simulink model "MIL_2018"  (R2018a)
settings: Solver=FixedStepDiscrete  StartTime=0.0  StopTime=49  FixedStep=1  MaxStep=1  RelTol=1e-3
undefined symbols (not defined in the file or in its folder): sigbuilder_block
settings Model: DataDictionary=Als_dd.sldd  Creator=Pratik shinde  LastModifiedBy=Pratik shinde
settings DataIOCC: ReturnWorkspaceOutputs=on
settings OptimizationCC: DefaultParameterBehavior=Inlined  EnhancedBackFolding=on  PassReuseOutputArgsAs=Individual arguments  ZeroExternalMemoryAtStartup=off  ZeroInternalMemoryAtStartup=off  OptimizeBlockOrder=speed  DifferentSizesBufferReuse=on  OptimizationCustomize=off
settings DebuggingCC: ParameterTunabilityLossMsg=error  ModelReferenceSymbolNameMessage=none
settings SFSimCC: SimUseLocalCustomCode=on  MATLABDynamicMemAlloc=off
settings RTWCC: SystemTargetFile=ert.tlc  GenCodeOnly=on  TemplateMakefile=ert_default_tmf  GenerateReport=on  RTWUseLocalCustomCode=on  IncludeHyperlinkInReport=on  LaunchReport=on  GenerateTraceInfo=on  GenerateTraceReport=on  GenerateTraceReportSl=on  GenerateTraceReportSf=on  GenerateTraceReportEml=on  GenerateWebview=on
settings CodeAppCC: ForceParamTrailComments=on  IgnoreCustomStorageClasses=off  OperatorAnnotations=on  SimulinkDataObjDesc=on  SFDataObjDesc=on  InsertBlockDesc=on
settings ERTTargetCC: TargetLangStandard=C99 (ISO)  GenerateSampleERTMain=on  InlinedParameterPlacement=NonHierarchical  ERTCustomFileTemplate=example_file_process.tlc
settings ConfigComp: CovMetricSettings=dcmw  CovHtmlReporting=on  DVTestSuiteOptimization=CombinedObjectives (Nonlinear Extended)  DVDetectOutOfBounds=on

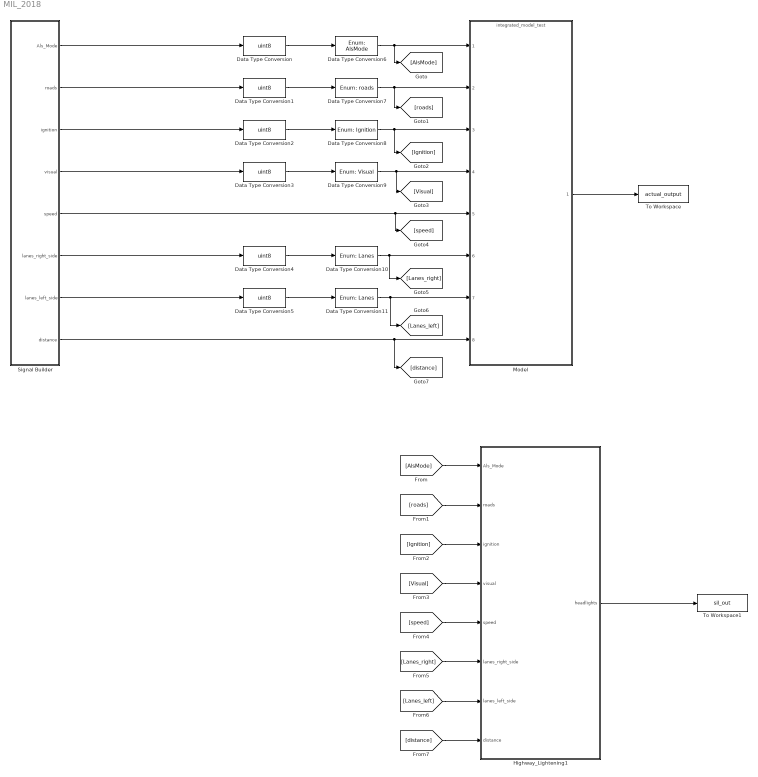
== system MIL_2018 ==
  Data Type Conversion{,1..5} (6 alike) : DataTypeConversion  OutDataTypeStr=uint8  SaturateOnIntegerOverflow=on  LockScale=on
  Data Type Conversion10 : DataTypeConversion  OutDataTypeStr=Enum: Lanes  SaturateOnIntegerOverflow=on  LockScale=on
  Data Type Conversion11 : DataTypeConversion  OutDataTypeStr=Enum: Lanes  SaturateOnIntegerOverflow=on  LockScale=on
  Data Type Conversion6 : DataTypeConversion  OutDataTypeStr=Enum: AlsMode  SaturateOnIntegerOverflow=on  LockScale=on
  Data Type Conversion7 : DataTypeConversion  OutDataTypeStr=Enum: roads  SaturateOnIntegerOverflow=on  LockScale=on
  Data Type Conversion8 : DataTypeConversion  OutDataTypeStr=Enum: Ignition  SaturateOnIntegerOverflow=on  LockScale=on
  Data Type Conversion9 : DataTypeConversion  OutDataTypeStr=Enum: Visual  SaturateOnIntegerOverflow=on  LockScale=on
  Highway_Lightening1 : Subsystem
      mask help: Simulink:masks:GenSFuncDesc_MD
      mask Help: eval('feval(''rtwprivate'',''rtwhelpview'',''rtw_sfcn_block'')');
  Model : ModelReference  ModelNameDialog=integrated_model_test.slx  SimulationMode=Normal  ModelReferenceVersion=1.36
  Signal Builder : Subsystem  Tag=STV Subsys  LoadFcn=sigbuilder_block('load');  StartFcn=sigbuilder_block('start');  StopFcn=sigbuilder_block('stop');  ClipboardFcn=sigbuilder_block('clipboard');  mask(Sigbuilder block){tuvar=[0:10]}
      mask help: Simulink:masks:SigbuilderBlock_MD
      mask init:
      | if ~strcmp(get_param(bdroot(gcbh),'SimulationStatus'),'stopped') tuvar = sigbuilder_block('maskInit'); end
      settings: CopyFcn=sigbuilder_block('copy');  DeleteFcn=sigbuilder_block('delete');  ModelCloseFcn=sigbuilder_block('modelClose');  PreSaveFcn=sigbuilder_block('preSave');  PauseFcn=sigbuilder_block('pause');  ContinueFcn=sigbuilder_block('continue');  NameChangeFcn=sigbuilder_block('namechange');  OpenFcn=sigbuilder_block('open',[437.6 199.2 550.4 400 ]);  CloseFcn=sigbuilder_block('close');
      mask Display: plot(0, 0, 100, 100,[2, 2, 32, 32, 2], [68, 8, 8, 68, 68],[32, 2], [38, 38], [32, 19, 2],[53, 60, 44], [32, 17, 17, 2],[16, 16, 31, 31]);txt = getActiveGroup(gcbh);text(2, 100, txt,'verticalAlignment', 'top');
  To Workspace : ToWorkspace  VariableName=actual_output  SaveFormat=Timeseries  SampleTime=-1
  To Workspace1 : ToWorkspace  VariableName=sil_out  SaveFormat=Timeseries  SampleTime=-1
  wires:
  Signal Builder/2(roads) -> Data Type Conversion1/1
  Signal Builder/3(ignition) -> Data Type Conversion2/1
  Signal Builder/4(visual) -> Data Type Conversion3/1
  Signal Builder/5(speed) -> [speed], Model/5
  Signal Builder/7(lanes_left_side) -> Data Type Conversion5/1
  Signal Builder/8(distance) -> [distance], Model/8
  Signal Builder/6(lanes_right_side) -> Data Type Conversion4/1
  Data Type Conversion/1 -> Data Type Conversion6/1
  Data Type Conversion1/1 -> Data Type Conversion7/1
  Data Type Conversion2/1 -> Data Type Conversion8/1
  Data Type Conversion3/1 -> Data Type Conversion9/1
  Data Type Conversion4/1 -> Data Type Conversion10/1
  Data Type Conversion5/1 -> Data Type Conversion11/1
  Data Type Conversion6/1 -> [AlsMode], Model/1
  Data Type Conversion7/1 -> [roads], Model/2
  Data Type Conversion8/1 -> [Ignition], Model/3
  Data Type Conversion9/1 -> [Visual], Model/4
  Data Type Conversion10/1 -> Model/6, [Lanes_right]
  Data Type Conversion11/1 -> Model/7, [Lanes_left]
  Model/1 -> To Workspace/1
  Signal Builder/1(Als_Mode) -> Data Type Conversion/1
  Highway_Lightening1/1(headlights) -> To Workspace1/1
  [AlsMode] -> Highway_Lightening1/1(Als_Mode)
  [roads] -> Highway_Lightening1/2(roads)
  [Ignition] -> Highway_Lightening1/3(ignition)
  [Visual] -> Highway_Lightening1/4(visual)
  [speed] -> Highway_Lightening1/5(speed)
  [Lanes_left] -> Highway_Lightening1/7(lanes_left_side)
  [distance] -> Highway_Lightening1/8(distance)
  [Lanes_right] -> Highway_Lightening1/6(lanes_right_side)

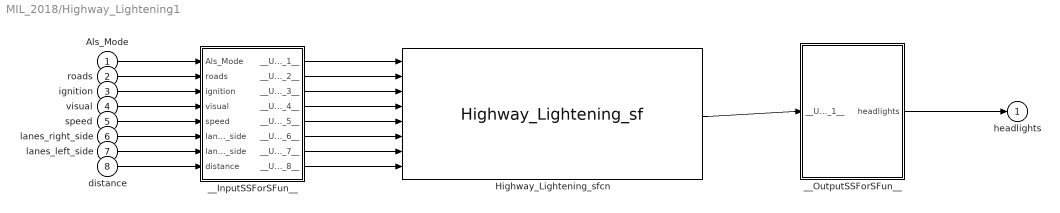
== system MIL_2018/Highway_Lightening1 ==
  Als_Mode : Inport
  roads : Inport  Port=2
  ignition : Inport  Port=3
  visual : Inport  Port=4
  speed : Inport  Port=5
  lanes_right_side : Inport  Port=6
  lanes_left_side : Inport  Port=7
  distance : Inport  Port=8
  Highway_Lightening_sfcn : S-Function  FunctionName=Highway_Lightening_sf  SFunctionModules=""  SFunctionDeploymentMode=off  EnableBusSupport=off  mask{rtw_sf_name=Highway_Lightening_sf, showVar=off}
      mask prompts: rtw_sf_name "Simulink:masks:GenSFuncName_MP"; showVar "Simulink:masks:GenSFuncShowModuleList_MP"
      mask help: Simulink:masks:GenSFuncDesc_MD
      mask init:
      | displist = '';
      | if ~strcmp(get_param(gcb, 'FunctionName'), rtw_sf_name);
      |   set_param(gcb, 'FunctionName', rtw_sf_name);
      | end
      | % Check if we are generating code
      | rtw_mode = false;
      | if strcmpi(get_param(bdroot(gcb),'SimulationStatus'),'Initializing')
      | 	rtw_mode = strcmpi(get_param(bdroot(gcb),'BuildingRTWCode'),'on') && ...
      | 		~strcmpi(get_param(bdroot(gcb),'TargetStyle'),'SimulationTarget');
      | end
      | if showVar || rtw_mode
      | 	if exist('rtwsfunc') == 2 | exist('rtwsfunc') == 6
      | 		tmplist = rtwsfunc(rtw_sf_name,gcb);
      | 		tmplist = DAStudio.message('Simulink:masks:GenSFuncListOfModules_IC', tmplist);
      | 	elseif showVar
      | 		tmplist1 = DAStudio.message('Simulink:masks:GenSFuncListOfModules_IC', '');
      |         tmplist2 = DAStudio.message('Simulink:masks:GenSFuncNotLicensed_IC');
      |         tmplist = [tmplist1 tmplist2];
      |  	end
      | end
      | if showVar
      |   displist = tmplist;
      | end
      settings: CopyFcn=|
      | if ~strcmp(get_param(gcb,'Linkstatus'),'none') && ...
      | ~strcmp(get_param(gcb,'Linkstatus'),'implicit')
      |   set_param(gcb,'LinkStatus','none');
      | end
      mask Help: eval('feval(''rtwprivate'',''rtwhelpview'',''rtw_sfcn_block'')');
      mask Display:
      | port_label('input',1,'Als_Mode');
      | port_label('input',2,'roads');
      | port_label('input',3,'ignition');
      | port_label('input',4,'visual');
      | port_label('input',5,'speed');
      | port_label('input',6,'lanes_right_side');
      | port_label('input',7,'lanes_left_side');
      | port_label('input',8,'distance');
      | port_label('output',1,'headlights');
  __InputSSForSFun__ : Subsystem
  __OutputSSForSFun__ : Subsystem
  headlights : Outport
  wires:
  __OutputSSForSFun__/1(headlights) -> headlights/1
  Highway_Lightening_sfcn/1 -> __OutputSSForSFun__/1(__UniqueInportName__1__)
  __InputSSForSFun__/8(__UniqueOutportName__8__) -> Highway_Lightening_sfcn/8
  __InputSSForSFun__/7(__UniqueOutportName__7__) -> Highway_Lightening_sfcn/7
  __InputSSForSFun__/6(__UniqueOutportName__6__) -> Highway_Lightening_sfcn/6
  __InputSSForSFun__/5(__UniqueOutportName__5__) -> Highway_Lightening_sfcn/5
  __InputSSForSFun__/4(__UniqueOutportName__4__) -> Highway_Lightening_sfcn/4
  __InputSSForSFun__/3(__UniqueOutportName__3__) -> Highway_Lightening_sfcn/3
  __InputSSForSFun__/2(__UniqueOutportName__2__) -> Highway_Lightening_sfcn/2
  __InputSSForSFun__/1(__UniqueOutportName__1__) -> Highway_Lightening_sfcn/1
  distance/1 -> __InputSSForSFun__/8(distance)
  lanes_left_side/1 -> __InputSSForSFun__/7(lanes_left_side)
  lanes_right_side/1 -> __InputSSForSFun__/6(lanes_right_side)
  speed/1 -> __InputSSForSFun__/5(speed)
  visual/1 -> __InputSSForSFun__/4(visual)
  ignition/1 -> __InputSSForSFun__/3(ignition)
  roads/1 -> __InputSSForSFun__/2(roads)
  Als_Mode/1 -> __InputSSForSFun__/1(Als_Mode)

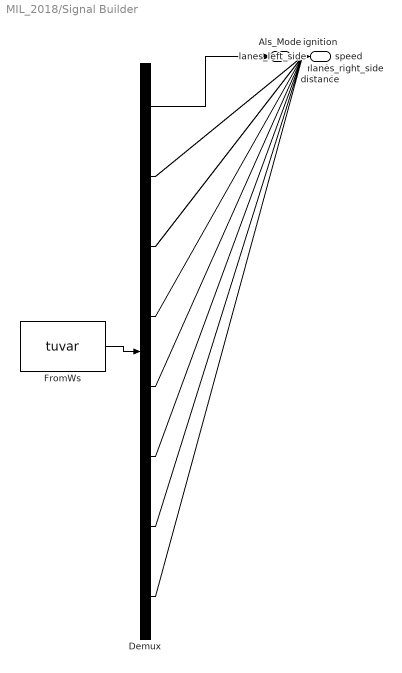
== system MIL_2018/Signal Builder ==
  Demux : Demux  Tag=STV Demux  Outputs=8
      settings: DisplayOption=none
  FromWs : FromWorkspace  Tag=STV FromWs  VariableName=tuvar
      SigBuilderData=|
      | common.afterFinalStr = 'Extrapolate'
      | common.sampleTime = 0
      | dataSet.timeRange = [0 10]
      | dataSet.name = 'Group 1'
      | sbobj.Groups.Name = 'Group 1'
      | sbobj.Groups.Signals(1).Name = 'Als_Mode'
      | sbobj.Groups.Signals(1).XData = [0 1 2 3 4 5 6 7 8 9 10 11 12 13 14 15 16 17 18 19 20 21 22 23 24 25 26 27 28 29 30 31 32 33 34 35 36 37 38 39 40 41 42 43 44 45 46 47 48 49]
      | sbobj.Groups.Signals(1).YData = [0 0 0 0 0 0 0 0 0 0 0 0 0 0 0 0 0 1 0 0 0 1 0 0 0 0 0 1 1 1 1 0 0 0 0 0 0 0 0 0 0 0 0 0 1 1 1 0 0 1]
      | sbobj.Groups.Signals(2).Name = 'roads'
      | sbobj.Groups.Signals(2).XData = [0 1 2 3 4 5 6 7 8 9 10 11 12 13 14 15 16 17 18 19 20 21 22 23 24 25 26 27 28 29 30 31 32 33 34 35 36 37 38 39 40 41 42 43 44 45 46 47 48 49]
      | sbobj.Groups.Signals(2).YData = [0 0 0 0 0 0 0 0 0 0 0 0 0 0 0 0 0 0 1 0 0 0 0 0 0 0 0 0 0 0 0 0 0 0 0 0 0 0 1 1 1 0 0 0 0 0 0 1 0 0]
      | sbobj.Groups.Signals(3).Name = 'ignition'
      | sbobj.Groups.Signals(3).XData = [0 1 2 3 4 5 6 7 8 9 10 11 12 13 14 15 16 17 18 19 20 21 22 23 24 25 26 27 28 29 30 31 32 33 34 35 36 37 38 39 40 41 42 43 44 45 46 47 48 49]
      | sbobj.Groups.Signals(3).YData = [0 0 0 0 0 0 0 0 0 0 0 0 0 0 0 0 0 0 0 1 0 0 0 0 1 1 1 0 0 0 0 0 0 0 0 0 0 0 0 0 0 1 1 1 1 1 1 0 1 0]
      | sbobj.Groups.Signals(4).Name = 'visual'
      | sbobj.Groups.Signals(4).XData = [0 1 2 3 4 5 6 7 8 9 10 11 12 13 14 15 16 17 18 19 20 21 22 23 24 25 26 27 28 29 30 31 32 33 34 35 36 37 38 39 40 41 42 43 44 45 46 47 48 49]
      | sbobj.Groups.Signals(4).YData = [1 1 1 1 1 1 1 1 1 1 1 1 1 1 1 1 1 1 1 1 0 0 0 0 0 0 0 1 1 1 0 1 1 1 1 1 1 1 1 1 1 1 1 1 1 1 1 1 1 1]
      | sbobj.Groups.Signals(5).Name = 'speed'
      | sbobj.Groups.Signals(5).XData = [0 1 2 3 4 5 6 7 8 9 10 11 12 13 14 15 16 17 18 19 20 21 22 23 24 25 26 27 28 29 30 31 32 33 34 35 36 37 38 39 40 41 42 43 44 45 46 47 48 49]
      | sbobj.Groups.Signals(5).YData = [125 100 125 125 125 125 125 125 90 125 125 125 125 125 125 125 125 125 125 125 125 100 125 100 100 125 125 125 125 125 125 100 125 125 125 125 125 100 125 125 125 125 125 125 125 125 125 125 125 125]
      | sbobj.Groups.Signals(6).Name = 'lanes_right_side'
      | sbobj.Groups.Signals(6).XData = [0 1 2 3 4 5 6 7 8 9 10 11 12 13 14 15 16 17 18 19 20 21 22 23 24 25 26 27 28 29 30 31 32 33 34 35 36 37 38 39 40 41 42 43 44 45 46 47 48 49]
      | sbobj.Groups.Signals(6).YData = [0 0 6 0 6 6 6 6 6 2 2 2 6 4 4 4 6 6 6 6 6 6 0 2 6 2 4 0 2 6 2 6 0 0 0 0 0 0 0 2 4 0 2 4 0 2 4 0 0 0]
      | sbobj.Groups.Signals(7).Name = 'lanes_left_side'
      | sbobj.Groups.Signals(7).XData = [0 1 2 3 4 5 6 7 8 9 10 11 12 13 14 15 16 17 18 19 20 21 22 23 24 25 26 27 28 29 30 31 32 33 34 35 36 37 38 39 40 41 42 43 44 45 46 47 48 49]
      | sbobj.Groups.Signals(7).YData = [6 6 6 1 1 1 1 1 1 6 6 6 3 6 6 6 5 5 5 5 5 1 6 6 1 3 5 6 3 1 3 6 6 6 1 1 1 1 1 3 5 1 3 5 1 3 5 1 1 1]
      | sbobj.Groups.Signals(8).Name = 'distance'
      | sbobj.Groups.Signals(8).XData = [0 1 2 3 4 5 6 7 8 9 10 11 12 13 14 15 16 17 18 19 20 21 22 23 24 25 26 27 28 29 30 31 32 33 34 35 36 37 38 39 40 41 42 43 44 45 46 47 48 49]
      | sbobj.Groups.Signals(8).YData = [25 25 25 25 9 35 25 20 20 25 10 55 25 35 25 75 35 35 35 35 35 35 40 35 55 35 25 25 35 45 45 0 9 40 25 9 35 9 25 30 35 25 30 35 25 30 35 35 35 35]
  Als_Mode : Outport  Tag=STV Outport
  roads : Outport  Tag=STV Outport  Port=2
  ignition : Outport  Tag=STV Outport  Port=3
  visual : Outport  Tag=STV Outport  Port=4
  speed : Outport  Tag=STV Outport  Port=5
  lanes_right_side : Outport  Tag=STV Outport  Port=6
  lanes_left_side : Outport  Tag=STV Outport  Port=7
  distance : Outport  Tag=STV Outport  Port=8
  wires:
  FromWs/1 -> Demux/1
  Demux/1 -> Als_Mode/1
  Demux/2 -> roads/1
  Demux/3 -> ignition/1
  Demux/4 -> visual/1
  Demux/5 -> speed/1
  Demux/6 -> lanes_right_side/1
  Demux/7 -> lanes_left_side/1
  Demux/8 -> distance/1

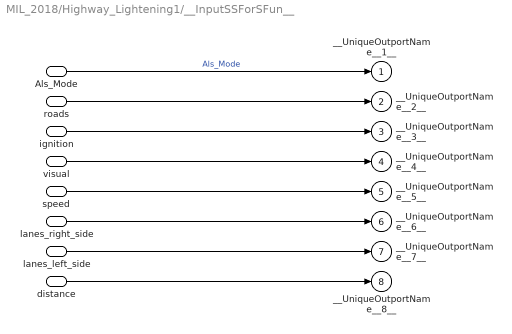
== system MIL_2018/Highway_Lightening1/__InputSSForSFun__ ==
  Als_Mode : Inport
  roads : Inport  Port=2
  ignition : Inport  Port=3
  visual : Inport  Port=4
  speed : Inport  Port=5
  lanes_right_side : Inport  Port=6
  lanes_left_side : Inport  Port=7
  distance : Inport  Port=8
  __UniqueOutportName__1__ : Outport
  __UniqueOutportName__2__ : Outport  Port=2
  __UniqueOutportName__3__ : Outport  Port=3
  __UniqueOutportName__4__ : Outport  Port=4
  __UniqueOutportName__5__ : Outport  Port=5
  __UniqueOutportName__6__ : Outport  Port=6
  __UniqueOutportName__7__ : Outport  Port=7
  __UniqueOutportName__8__ : Outport  Port=8
  wires:
  distance/1 -> __UniqueOutportName__8__/1
  lanes_left_side/1 -> __UniqueOutportName__7__/1
  lanes_right_side/1 -> __UniqueOutportName__6__/1
  speed/1 -> __UniqueOutportName__5__/1
  visual/1 -> __UniqueOutportName__4__/1
  ignition/1 -> __UniqueOutportName__3__/1
  roads/1 -> __UniqueOutportName__2__/1
  Als_Mode/1 -> __UniqueOutportName__1__/1  "Als_Mode"

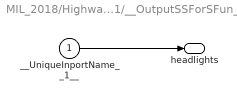
== system MIL_2018/Highway_Lightening1/__OutputSSForSFun__ ==
  __UniqueInportName__1__ : Inport
  headlights : Outport
  wires:
  __UniqueInportName__1__/1 -> headlights/1
